simulink model "feeder_1_1_sm_feeder1"  (Simulink 9.2)
settings: Solver=ode4  StartTime=0.0  StopTime=inf  FixedStep=0.0001  RelTol=1e-3
PreLoadFcn:
  | Ts=100e-6;Core_Num = 0;
PostLoadFcn:
  | Ts=100e-6;Core_Num = 0;
InitFcn:
  | Ts=100e-6;Core_Num = 0;
undefined symbols (not defined in the file or in its folder): another_event_name, D11, Delta, my_event_name
libraries: powerlib x91, powerlib_meascontrol x28, simulink x9, opal_lib x3, artemis x2, rtio_generic_ethernet x1, rtio_opalrt_ml605ex1 x1, rtlab x1, rtio_spectracom x1
(part 1 of 2)
settings Model: ARTEMISmethode_block_infos=$$__separator__$$feeder_1_1_sm_feeder1/ARTEMIS Guide1$$__separator__$$  Creator=DETLDAQ  LastModifiedBy=DETLDAQ
settings OptimizationCC: BlockReduction=off  BooleanDataType=off  OptimizeBlockIOStorage=off  BufferReuse=off  GlobalBufferReuse=off  ExpressionFolding=off  LocalBlockOutputs=off  OptimizeDataStoreBuffers=off  BusAssignmentInplaceUpdate=off
settings DebuggingCC: SaveWithParameterizedLinksMsg=none  SignalResolutionControl=TryResolveAllWithWarning  MultiTaskDSMMsg=warning  MultiTaskCondExecSysMsg=none  FcnCallInpInsideContextMsg=error
settings HardwareCC: TargetUnknown=on
settings RTWCC: GenCodeOnly=on
settings GRTTargetCC: CombineOutputUpdateFcns=on  GRTInterface=off
settings SimscapeCC: SimscapeNormalizeSystem=off

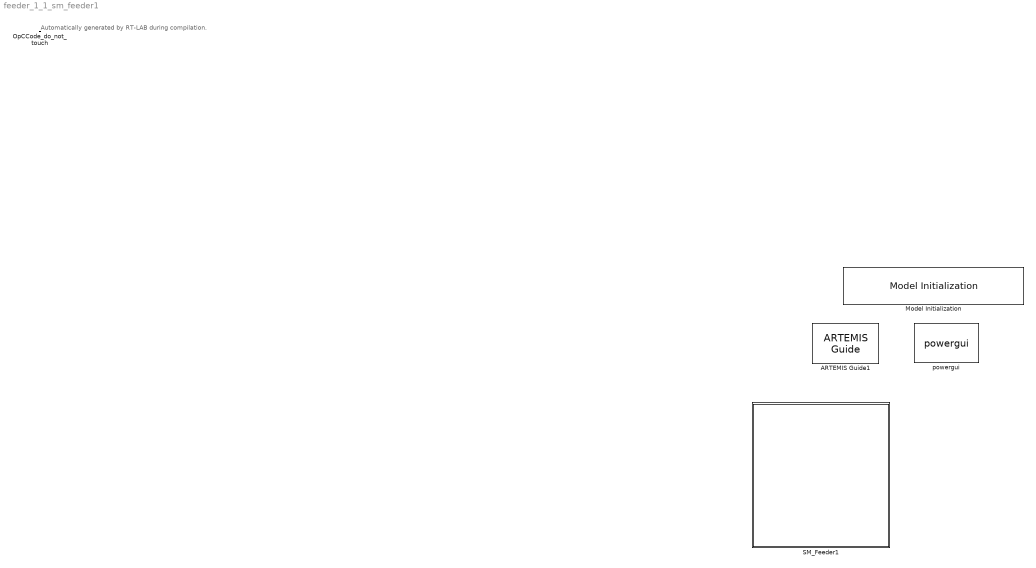
== system feeder_1_1_sm_feeder1 ==
  note: Automatically generated by RT-LAB during compilation.
  ARTEMIS Guide1 : artemis/ARTEMIS/ARTEMIS Guide  Tag=FTSSmethode_opal_4hx0r99  Description=5.0_z1  lock=on  Ts=Ts  opt=art5  dyna=off  nb_perm=4  RT_fullcomp=off  ssn=on  ssn_itvc=off  ssn_ivic=off  ssn_ext=off  ssn_solver=Backward Euler  ssn_impulse=off  ssn_quasimpulse=off  ssn_impulse_loop=5  paraExtinctionThy=off  Thy_Impulse=off  dtc=Off  dtc_opt=normal  ao=on  simtype=off  ct_mac=off  lin_mov=off  lsp=[0.001 2]  spike_skip=Disabled  dtc_extra=1  dtc_sws=normal  dtc_pied=0.5  SPSRulesBlock=SPSRules  tre=off  ctmm=off  LF=on  dpl_type=ARTEMiS DPL  rlc_type=off  custom_type=off  para=on  ssn_ImpulseLoopBlockedStateUpdate=5  ssn_mov_iter_number=5  ssn_switch_iter_number=5  ssn_nib_type_verify=on  ssn_use_lu=on  ssn_use_ldlt=off
  Model Initialization : artemis/Tools /Misc/Model Initialization  InitFcnX=Ts=100e-6;Core_Num = 0;  prel=on  posl=on  inif=on  strf=off
  OpCCode_do_not_touch : opal_lib/Communication/OpCCode  SystemSampleTime=-1
  SM_Feeder1 : Subsystem
  powergui : powerlib/powergui  SimulationMode=Discrete  SampleTime=0.0001  frequency=60  Iterations=50  frequencyindice=0  Pbase=100e6  ErrMax=0.0001  UnitsV=kV  UnitsW=MW  buscounter=0  FunctionMessages=off  echomessages=off  EnableUseOfTLC=off  CurrentSourceSwitches=off  DisableSnubberDevices=off  DisableRonSwitches=off  DisableVfSwitches=off  DisplayEquations=off  SolverType=Backward Euler  Interpol=off  ExternalGateDelay=off  methode=off  Ts=100  x0status=blocks  SPID=off  SwTol=0  HookPort=off  RestoreLinks=warning  ResistiveCurrentMeasurement=off  Frange=[0:2:500]  Ylog=off  Xlog=on  ShowGrid=off  save=off  variable=ZData  structure=0  ZoomFFT=off  StartTime=0.0  cycles=1  DisplayStyle=1  fundamental=60  FreqAxis=off  MaxFrequency=1000  frequencyindicesteady=1  RmsSteady=1  display=off

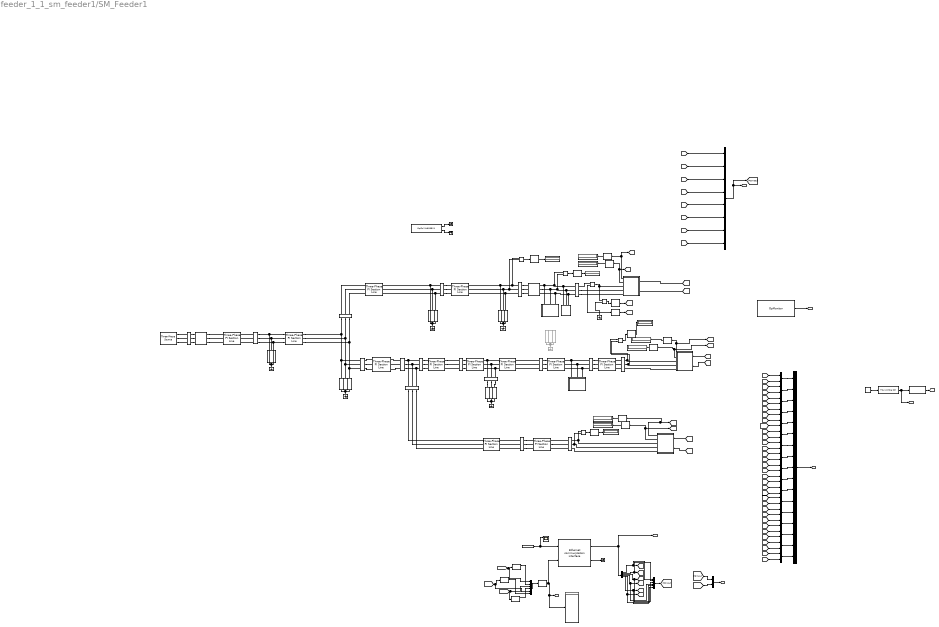
== system feeder_1_1_sm_feeder1/SM_Feeder1 ==
  note: included
  note: Included
  note: Included in SE
  note: Not include
  note: Not include in SE
  note: not include in SE
  Auxiliary Load : powerlib/Elements/Three-Phase Parallel RLC Load  LConnTagsString=A|B|C  Configuration=Y (grounded)  NominalVoltage=480  Vabc=[1e3 1e3 1e3]  Vabcp=[1e3 1e3 1e3]  NominalFrequency=60  UnbalancedPower=off  ActivePower=1  InductivePower=0  CapacitivePower=0  Pabc=[10e3 9e3 11e3]  QLabc=[100 90 110]  QCabc=[100 90 110]  Pabcp=[10e3 9e3 11e3]  QLabcp=[100 90 110]  QCabcp=[100 90 110]  Measurements=None  LoadType=constant Z
  Bus Creator : BusCreator  Inputs=17
  Constant8 : Constant
  Current Measurement : powerlib/Measurements/Current Measurement  PhasorSimulation=off  OutputType=Complex  PSBequivalent=0
  Demux1 : Demux  Outputs=6
  Display{,1,4..9,15..16} (10 alike) : Display
      Display15 settings: Format=bank
      Display4 settings: Format=bank
      Display5 settings: Format=bank
      Display7 settings: Format=bank
      Display8 settings: Format=bank
  Dynamic Load BCDC : Subsystem
  Dynamic Load Landfill : Subsystem
  Ethernet communication interface : rtio_generic_ethernet/Ethernet communication interface  ctrl_id=1  nbr_to_remote_endpoint=12  type_to_remote_endpoint=FLOAT  offset_to_remote_endpoint=0  swap_tx=on  nbr_from_remote_endpoint=6  type_from_remote_endpoint=FLOAT  offset_from_remote_endpoint=0  swap_rx=on  exe_name='AsyncEthernet'  nic_name='eth0'  protocol=TCP  tcp_mode=Client  port=6340  remote_ip='10.1.2.2'
  Ground{1..3,5,7..8} (6 alike) : powerlib/Elements/Ground  LConnTagsString=a
  Ground4 : powerlib/Elements/Ground  Commented=on  LConnTagsString=a
  IED1 : powerlib/Measurements/Three-Phase V-I Measurement  VoltageMeasurement=phase-to-ground  SetLabelV=on  LabelV=V_IED1  Vpu=off  VpuLL=off  CurrentMeasurement=yes  SetLabelI=on  LabelI=I_IED1  Ipu=off  Pbase=100e6  Vbase=500e3  OutputType=Complex  PhasorSimulation=off  PSBequivalent=0
  IED10 : powerlib/Measurements/Three-Phase V-I Measurement  VoltageMeasurement=phase-to-ground  SetLabelV=on  LabelV=V_IED10  Vpu=off  VpuLL=off  CurrentMeasurement=yes  SetLabelI=on  LabelI=I_IED10  Ipu=off  Pbase=100e6  Vbase=500e3  OutputType=Complex  PhasorSimulation=off  PSBequivalent=0
  IED11 : powerlib/Measurements/Three-Phase V-I Measurement  VoltageMeasurement=phase-to-ground  SetLabelV=on  LabelV=V_IED11  Vpu=off  VpuLL=off  CurrentMeasurement=yes  SetLabelI=on  LabelI=I_IED11  Ipu=off  Pbase=100e6  Vbase=500e3  OutputType=Complex  PhasorSimulation=off  PSBequivalent=0
  IED12 : powerlib/Measurements/Three-Phase V-I Measurement  VoltageMeasurement=phase-to-ground  SetLabelV=on  LabelV=V_IED12  Vpu=off  VpuLL=off  CurrentMeasurement=yes  SetLabelI=on  LabelI=I_IED12  Ipu=off  Pbase=100e6  Vbase=500e3  OutputType=Complex  PhasorSimulation=off  PSBequivalent=0
  IED13 : powerlib/Measurements/Three-Phase V-I Measurement  VoltageMeasurement=phase-to-ground  SetLabelV=on  LabelV=V_IED13  Vpu=off  VpuLL=off  CurrentMeasurement=yes  SetLabelI=on  LabelI=I_IED13  Ipu=off  Pbase=100e6  Vbase=500e3  OutputType=Complex  PhasorSimulation=off  PSBequivalent=0
  IED14 : powerlib/Measurements/Three-Phase V-I Measurement  VoltageMeasurement=phase-to-ground  SetLabelV=on  LabelV=V_IED14  Vpu=off  VpuLL=off  CurrentMeasurement=yes  SetLabelI=on  LabelI=I_IED14  Ipu=off  Pbase=100e6  Vbase=500e3  OutputType=Complex  PhasorSimulation=off  PSBequivalent=0
  IED15 : powerlib/Measurements/Three-Phase V-I Measurement  VoltageMeasurement=phase-to-ground  SetLabelV=on  LabelV=V_IED15  Vpu=off  VpuLL=off  CurrentMeasurement=yes  SetLabelI=on  LabelI=I_IED15  Ipu=off  Pbase=100e6  Vbase=500e3  OutputType=Complex  PhasorSimulation=off  PSBequivalent=0
  IED16 : powerlib/Measurements/Three-Phase V-I Measurement  VoltageMeasurement=phase-to-ground  SetLabelV=on  LabelV=V_IED16  Vpu=off  VpuLL=off  CurrentMeasurement=yes  SetLabelI=on  LabelI=I_IED16  Ipu=off  Pbase=100e6  Vbase=500e3  OutputType=Complex  PhasorSimulation=off  PSBequivalent=0
  IED17 : powerlib/Measurements/Three-Phase V-I Measurement  VoltageMeasurement=phase-to-ground  SetLabelV=on  LabelV=V_IED17  Vpu=off  VpuLL=off  CurrentMeasurement=yes  SetLabelI=on  LabelI=I_IED17  Ipu=off  Pbase=100e6  Vbase=500e3  OutputType=Complex  PhasorSimulation=off  PSBequivalent=0
  IED2 : powerlib/Measurements/Three-Phase V-I Measurement  VoltageMeasurement=phase-to-ground  SetLabelV=on  LabelV=V_IED2  Vpu=off  VpuLL=off  CurrentMeasurement=yes  SetLabelI=on  LabelI=I_IED2  Ipu=off  Pbase=100e6  Vbase=500e3  OutputType=Complex  PhasorSimulation=off  PSBequivalent=0
  IED3 : powerlib/Measurements/Three-Phase V-I Measurement  VoltageMeasurement=phase-to-ground  SetLabelV=on  LabelV=V_IED3  Vpu=off  VpuLL=off  CurrentMeasurement=yes  SetLabelI=on  LabelI=I_IED3  Ipu=off  Pbase=100e6  Vbase=500e3  OutputType=Complex  PhasorSimulation=off  PSBequivalent=0
  IED4 : powerlib/Measurements/Three-Phase V-I Measurement  VoltageMeasurement=phase-to-ground  SetLabelV=on  LabelV=V_IED4  Vpu=off  VpuLL=off  CurrentMeasurement=yes  SetLabelI=on  LabelI=I_IED4  Ipu=off  Pbase=100e6  Vbase=500e3  OutputType=Complex  PhasorSimulation=off  PSBequivalent=0
  IED5 : powerlib/Measurements/Three-Phase V-I Measurement  VoltageMeasurement=phase-to-ground  SetLabelV=on  LabelV=V_IED5  Vpu=off  VpuLL=off  CurrentMeasurement=yes  SetLabelI=on  LabelI=I_IED5  Ipu=off  Pbase=100e6  Vbase=500e3  OutputType=Complex  PhasorSimulation=off  PSBequivalent=0
  IED6 : powerlib/Measurements/Three-Phase V-I Measurement  VoltageMeasurement=phase-to-ground  SetLabelV=on  LabelV=V_IED6  Vpu=off  VpuLL=off  CurrentMeasurement=yes  SetLabelI=on  LabelI=I_IED6  Ipu=off  Pbase=100e6  Vbase=500e3  OutputType=Complex  PhasorSimulation=off  PSBequivalent=0
  IED7 : powerlib/Measurements/Three-Phase V-I Measurement  VoltageMeasurement=phase-to-ground  SetLabelV=on  LabelV=V_IED7  Vpu=off  VpuLL=off  CurrentMeasurement=yes  SetLabelI=on  LabelI=I_IED7  Ipu=off  Pbase=100e6  Vbase=500e3  OutputType=Complex  PhasorSimulation=off  PSBequivalent=0
  IED8 : powerlib/Measurements/Three-Phase V-I Measurement  VoltageMeasurement=phase-to-ground  SetLabelV=on  LabelV=V_IED8  Vpu=off  VpuLL=off  CurrentMeasurement=yes  SetLabelI=on  LabelI=I_IED8  Ipu=off  Pbase=100e6  Vbase=500e3  OutputType=Complex  PhasorSimulation=off  PSBequivalent=0
  IED9 : powerlib/Measurements/Three-Phase V-I Measurement  VoltageMeasurement=phase-to-ground  SetLabelV=on  LabelV=V_IED9  Vpu=off  VpuLL=off  CurrentMeasurement=yes  SetLabelI=on  LabelI=I_IED9  Ipu=off  Pbase=100e6  Vbase=500e3  OutputType=Complex  PhasorSimulation=off  PSBequivalent=0
  Line105 : powerlib/Elements/Three-Phase PI Section Line  LConnTagsString=a|b|c  RConnTagsString=A|B|C  Frequency=60  Resistances=[0.713799213 1.084564961]  Inductances=[0.001374518 0.004235717]  Capacitances=[1.12126E-07 1.12126E-07]  Length=3.436427976
      settings: SourceProductName=Simscape Power Systems
  Line135 : powerlib/Elements/Three-Phase PI Section Line  LConnTagsString=a|b|c  RConnTagsString=A|B|C  Frequency=60  Resistances=[0.437335958 0.80347769]  Inductances=[ 0.00135414 0.00422516]  Capacitances=[1.12126E-07 1.12126E-07]  Length=0.054899113
      settings: SourceProductName=Simscape Power Systems
  Line149 : powerlib/Elements/Three-Phase PI Section Line  LConnTagsString=a|b|c  RConnTagsString=A|B|C  Frequency=60  Resistances=[0.080380577 0.200459318]  Inductances=[0.000297632 0.000175795]  Capacitances=[1.12126E-07 1.12126E-07]  Length=0.001045348
      settings: SourceProductName=Simscape Power Systems
  Line150 : powerlib/Elements/Three-Phase PI Section Line  LConnTagsString=a|b|c  RConnTagsString=A|B|C  Frequency=60  Resistances=[0.076844259 0.363286089]  Inductances=[0.000938984 0.003273312]  Capacitances=[1.12126E-07 1.12126E-07]  Length=3.569857224
      settings: SourceProductName=Simscape Power Systems
  Line164 : powerlib/Elements/Three-Phase PI Section Line  LConnTagsString=a|b|c  RConnTagsString=A|B|C  Frequency=60  Resistances=[0.104986877 0.326771654]  Inductances=[0.000315038 0.000223659]  Capacitances=[1.12126E-07 1.12126E-07]  Length=0.024037250
      settings: SourceProductName=Simscape Power Systems
  Line167 : powerlib/Elements/Three-Phase PI Section Line  LConnTagsString=a|b|c  RConnTagsString=A|B|C  Frequency=60  Resistances=[0.146325459 0.420275591]  Inductances=[0.001054767 0.003564625]  Capacitances=[1.12126E-07 1.12126E-07]  Length=0.039662466
      settings: SourceProductName=Simscape Power Systems
  Line188 : powerlib/Elements/Three-Phase PI Section Line  LConnTagsString=a|b|c  RConnTagsString=A|B|C  Frequency=60  Resistances=[0.074475066 0.348425197]  Inductances=[0.000982535 0.003492392]  Capacitances=[1.12126E-07 1.12126E-07]  Length=0.354198631
      settings: SourceProductName=Simscape Power Systems
  Line196 : powerlib/Elements/Three-Phase PI Section Line  LConnTagsString=a|b|c  RConnTagsString=A|B|C  Frequency=60  Resistances=[0.1820739 0.3053387]  Inductances=[0.000581495 0.000514283]  Capacitances=[3.41761e-8 3.4176e-8]  Length=0.029452870
      settings: SourceProductName=Simscape Power Systems
  Line4 : powerlib/Elements/Three-Phase PI Section Line  LConnTagsString=a|b|c  RConnTagsString=A|B|C  Frequency=60  Resistances=[8.150387E-02 0.348876969]  Inductances=[0.000906839 0.003088814]  Capacitances=[1.12126E-07 1.12126E-07]  Length=0.314096400
      settings: SourceProductName=Simscape Power Systems
  Line59 : powerlib/Elements/Three-Phase PI Section Line  LConnTagsString=a|b|c  RConnTagsString=A|B|C  Frequency=60  Resistances=[0.074475066 0.348425197]  Inductances=[0.000982535 0.003492393]  Capacitances=[1.12126E-07 1.12126E-07]  Length=1.094945842
      settings: SourceProductName=Simscape Power Systems
  Line88 : powerlib/Elements/Three-Phase PI Section Line  LConnTagsString=a|b|c  RConnTagsString=A|B|C  Frequency=60  Resistances=[7.447507E-02 0.348425197]  Inductances=[0.000982535 0.003492393]  Capacitances=[1.12126E-07 1.12126E-07]  Length=0.079929441
      settings: SourceProductName=Simscape Power Systems
  Line97 : powerlib/Elements/Three-Phase PI Section Line  LConnTagsString=a|b|c  RConnTagsString=A|B|C  Frequency=60  Resistances=[7.447507E-02 0.348425197]  Inductances=[0.000982535 0.003492393]  Capacitances=[1.12126E-07 1.12126E-07]  Length=0.080325681
      settings: SourceProductName=Simscape Power Systems
  Mux{1,3..4,6..19,34} (18 alike) : Mux  Inputs=2
  Mux2 : Mux  Inputs=8
  Mux20 : Mux  Inputs=6
  Mux5 : Mux  Inputs=6
  OpCtrl ML605EX1 : rtio_opalrt_ml605ex1/OpCtrl ML605EX1  CtrlName='ML605EX1 Ctrl'  boardid=0  BitstreamFilename=ML605_2-EX-0029-2_2_6_61-32Aio_32DioSelectable-01-01.bin  numconfig=-1  mode=Master  externalClock=off  decimRtsi=0  calibIO=off  SampleTime=0  loadinport=-1
  OpMonitor : rtlab/Monitoring/OpMonitor  compute_time=off  real_step=off  idle_time=off  nb_overruns=on  user_time=off  user_name=my_event_name,another_event_name
  PLL (3ph) : powerlib_meascontrol/PLL/PLL (3ph)  Fmin=45  Par_Init=[0, 60]  ParK=[180, 3200, 1]  TcD=1e-4  MaxRateChangeFreq=12  FilterCutOffFreq=25  Ts=0  AGC=on
  PLL (3ph)1 : powerlib_meascontrol/PLL/PLL (3ph)  Fmin=45  Par_Init=[0, 60]  ParK=[180, 3200, 1]  TcD=1e-4  MaxRateChangeFreq=12  FilterCutOffFreq=25  Ts=0  AGC=on
  PLL (3ph)2 : powerlib_meascontrol/PLL/PLL (3ph)  Fmin=45  Par_Init=[0, 60]  ParK=[180, 3200, 1]  TcD=1e-4  MaxRateChangeFreq=12  FilterCutOffFreq=25  Ts=0  AGC=on
  PLL power injector : Subsystem  mask{ratedP=258*1000, ratedV=480, KP_I=2, KI_I=20, Res=0.00893, Ind=1.895e-3}
      mask prompts: ratedP "Rated Power (VA)"; ratedV "Rated Voltage (Vrms)"; KP_I "KP of Current Regulator"; KI_I "KI of current regulator"; Res "Ri (ohms)"; Ind "Li (Henrys)"
      mask init:
      | Sb = ratedP;
      | Vb = ratedV*sqrt(2)/sqrt(3);
      | Wb = 2*pi*60;
      | Ib = Sb*sqrt(2)/ratedV/sqrt(3);
      | Zb = Vb/Ib;
      | Lb = Zb/Wb;
      | 
      | Ri = Res;
      | Li = Ind;
      | Ri_pu = Ri/Zb;
      | Li_pu = Li/Lb;
      | 
      | KP = KP_I;
      | KI = KI_I;
  PLL power injector1 : Subsystem  mask{ratedP=10000000, ratedV=12470, KP_I=2, KI_I=20, Res=0.01555, Ind=3.3e-3}
      mask prompts: ratedP "Rated Power (VA)"; ratedV "Rated Voltage (Vrms)"; KP_I "KP of Current Regulator"; KI_I "KI of current regulator"; Res "Ri (ohms)"; Ind "Li (Henrys)"
      mask init:
      | Sb = ratedP;
      | Vb = ratedV*sqrt(2)/sqrt(3);
      | Wb = 2*pi*60;
      | Ib = Sb*sqrt(2)/ratedV/sqrt(3);
      | Zb = Vb/Ib;
      | Lb = Zb/Wb;
      | 
      | Ri = Res;
      | Li = Ind;
      | Ri_pu = Ri/Zb;
      | Li_pu = Li/Lb;
      | 
      | KP = KP_I;
      | KI = KI_I;
  PLL power injector2 : Subsystem  mask{ratedP=10000000, ratedV=12470, KP_I=2, KI_I=20, Res=0.1555, Ind=0.033}
      mask prompts: ratedP "Rated Power (VA)"; ratedV "Rated Voltage (Vrms)"; KP_I "KP of Current Regulator"; KI_I "KI of current regulator"; Res "Ri (ohms)"; Ind "Li (Henrys)"
      mask init:
      | Sb = ratedP;
      | Vb = ratedV*sqrt(2)/sqrt(3);
      | Wb = 2*pi*60;
      | Ib = Sb*sqrt(2)/ratedV/sqrt(3);
      | Zb = Vb/Ib;
      | Lb = Zb/Wb;
      | 
      | Ri = Res;
      | Li = Ind;
      | Ri_pu = Ri/Zb;
      | Li_pu = Li/Lb;
      | 
      | KP = KP_I;
      | KI = KI_I;
  Pulse input : DiscretePulseGenerator  Period=round(1/Ts)  SampleTime=Ts
  RMS{,1..6,11..15} (12 alike) : powerlib_meascontrol/Measurements/RMS  TrueRMS=on  Freq=60  RMSInit=120  Ts=Ts
  RMS28 : powerlib_meascontrol/Measurements/RMS  TrueRMS=on  Freq=60  RMSInit=480  Ts=Ts
  Scope : Scope  NumInputPorts=2
  Series  Load1 : powerlib/Elements/Series RLC Load  LConnTagsString=a  RConnTagsString=__new0  NominalVoltage=7199.557857  NominalFrequency=60  ActivePower=2670.415479  InductivePower=302.451287  CapacitivePower=0  Setx0=off  InitialVoltage=0  SetiL0=off  InitialCurrent=0  Measurements=None  LoadType=constant PQ
  Series  Load10 : powerlib/Elements/Series RLC Load  Commented=on  LConnTagsString=a  RConnTagsString=__new0  NominalVoltage=480  NominalFrequency=60  ActivePower=25500  InductivePower=19200  CapacitivePower=0  Setx0=off  InitialVoltage=0  SetiL0=off  InitialCurrent=0  Measurements=None  LoadType=constant PQ
  Series  Load11 : powerlib/Elements/Series RLC Load  Commented=on  LConnTagsString=a  RConnTagsString=__new0  NominalVoltage=480  NominalFrequency=60  ActivePower=25500  InductivePower=19200  CapacitivePower=0  Setx0=off  InitialVoltage=0  SetiL0=off  InitialCurrent=0  Measurements=None  LoadType=constant PQ
  Series  Load12 : powerlib/Elements/Series RLC Load  Commented=on  LConnTagsString=a  RConnTagsString=__new0  NominalVoltage=480  NominalFrequency=60  ActivePower=25500  InductivePower=19200  CapacitivePower=0  Setx0=off  InitialVoltage=0  SetiL0=off  InitialCurrent=0  Measurements=None  LoadType=constant PQ
  Series  Load13 : powerlib/Elements/Series RLC Load  LConnTagsString=a  RConnTagsString=__new0  NominalVoltage=7199.557857  NominalFrequency=60  ActivePower=118930.1571  InductivePower=12605.38342  CapacitivePower=0  Setx0=off  InitialVoltage=0  SetiL0=off  InitialCurrent=0  Measurements=None  LoadType=constant PQ
  Series  Load14 : powerlib/Elements/Series RLC Load  LConnTagsString=a  RConnTagsString=__new0  NominalVoltage=7199.557857  NominalFrequency=60  ActivePower=107384.1981  InductivePower=11558.83111  CapacitivePower=0  Setx0=off  InitialVoltage=0  SetiL0=off  InitialCurrent=0  Measurements=None  LoadType=constant PQ
  Series  Load15 : powerlib/Elements/Series RLC Load  LConnTagsString=a  RConnTagsString=__new0  NominalVoltage=7199.557857  NominalFrequency=60  ActivePower=108561.8938  InductivePower=11911.28039  CapacitivePower=0  Setx0=off  InitialVoltage=0  SetiL0=off  InitialCurrent=0  Measurements=None  LoadType=constant PQ
  Series  Load16 : powerlib/Elements/Series RLC Load  LConnTagsString=a  RConnTagsString=__new0  NominalVoltage=7199.557857  NominalFrequency=60  ActivePower=116317.6881  InductivePower=25615.54001  CapacitivePower=0  Setx0=off  InitialVoltage=0  SetiL0=off  InitialCurrent=0  Measurements=None  LoadType=constant PQ
  Series  Load17 : powerlib/Elements/Series RLC Load  LConnTagsString=a  RConnTagsString=__new0  NominalVoltage=7199.557857  NominalFrequency=60  ActivePower=97118.47107  InductivePower=22060.3874  CapacitivePower=0  Setx0=off  InitialVoltage=0  SetiL0=off  InitialCurrent=0  Measurements=None  LoadType=constant PQ
  Series  Load18 : powerlib/Elements/Series RLC Load  LConnTagsString=a  RConnTagsString=__new0  NominalVoltage=7199.557857  NominalFrequency=60  ActivePower=100579.6302  InductivePower=22407.05615  CapacitivePower=0  Setx0=off  InitialVoltage=0  SetiL0=off  InitialCurrent=0  Measurements=None  LoadType=constant PQ
  Series  Load19 : powerlib/Elements/Series RLC Load  LConnTagsString=a  RConnTagsString=__new0  NominalVoltage=12470  NominalFrequency=60  ActivePower=0  InductivePower=0  CapacitivePower=1800000  Setx0=off  InitialVoltage=0  SetiL0=off  InitialCurrent=0  Measurements=None  LoadType=constant Z
  Series  Load2 : powerlib/Elements/Series RLC Load  LConnTagsString=a  RConnTagsString=__new0  NominalVoltage=7199.557857  NominalFrequency=60  ActivePower=0  InductivePower=3.438665  CapacitivePower=0  Setx0=off  InitialVoltage=0  SetiL0=off  InitialCurrent=0  Measurements=None  LoadType=constant PQ
  Series  Load20 : powerlib/Elements/Series RLC Load  LConnTagsString=a  RConnTagsString=__new0  NominalVoltage=12470  NominalFrequency=60  ActivePower=0  InductivePower=0  CapacitivePower=1800000  Setx0=off  InitialVoltage=0  SetiL0=off  InitialCurrent=0  Measurements=None  LoadType=constant Z
  Series  Load21 : powerlib/Elements/Series RLC Load  LConnTagsString=a  RConnTagsString=__new0  NominalVoltage=12470  NominalFrequency=60  ActivePower=0  InductivePower=0  CapacitivePower=1800000  Setx0=off  InitialVoltage=0  SetiL0=off  InitialCurrent=0  Measurements=None  LoadType=constant Z
  Series  Load3 : powerlib/Elements/Series RLC Load  LConnTagsString=a  RConnTagsString=__new0  NominalVoltage=7199.557857  NominalFrequency=60  ActivePower=3860.344758  InductivePower=489.471522  CapacitivePower=0  Setx0=off  InitialVoltage=0  SetiL0=off  InitialCurrent=0  Measurements=None  LoadType=constant PQ
  Series  Load4 : powerlib/Elements/Series RLC Load  LConnTagsString=a  RConnTagsString=__new0  NominalVoltage=7199.557857  NominalFrequency=60  ActivePower=393.998726  InductivePower=154.409997  CapacitivePower=0  Setx0=off  InitialVoltage=0  SetiL0=off  InitialCurrent=0  Measurements=None  LoadType=constant PQ
  Series  Load5 : powerlib/Elements/Series RLC Load  LConnTagsString=a  RConnTagsString=__new0  NominalVoltage=7199.557857  NominalFrequency=60  ActivePower=28.182185  InductivePower=0  CapacitivePower=8.948845  Setx0=off  InitialVoltage=0  SetiL0=off  InitialCurrent=0  Measurements=None  LoadType=constant PQ
  Series  Load6 : powerlib/Elements/Series RLC Load  LConnTagsString=a  RConnTagsString=__new0  NominalVoltage=7199.557857  NominalFrequency=60  ActivePower=2288.289329  InductivePower=413.71859  CapacitivePower=0  Setx0=off  InitialVoltage=0  SetiL0=off  InitialCurrent=0  Measurements=None  LoadType=constant PQ
  TSync PCIe Ctrl1 : rtio_spectracom/TSync PCIe Ctrl  devIx=0  holdover_timeout=5  timestamp_en=on  set_time_en=off  ts_wo_sync_opt=Simulation time
  Terminator1 : Terminator
  Terminator2 : Terminator
  Terminator3 : Terminator
  Three-Phase Transformer (Two Windings) : powerlib/Elements/Three-Phase Transformer (Two Windings)  Winding1Connection=Delta (D11)  Winding2Connection=Yg  CoreType=Three single-phase transformers  SetSaturation=off  Hysteresis=off  DataFile='hysteresis'  SetInitialFlux=off  Measurements=None  UNITS=pu  NominalPower=[30000e3 , 60 ]  Winding1=[ 115e3 , 0.0005 , 0.07755]  Winding2=[ 12.47e3, 0.0005 ,0.07755 ]  Rm=200  Lm=200  L0=0.5  Saturation=[ 0,0 ; 0.0024,1.2 ; 1.0,1.52 ]  InitialFluxes=[ 0.8 , -0.8 , 0.7 ]  MoreParameters=off  BreakLoop=off  DataType=off  TransfoNumber=1
  Three-Phase Transformer (Two Windings)5 : powerlib/Elements/Three-Phase Transformer (Two Windings)  Winding1Connection=Yg  Winding2Connection=Yg  CoreType=Three single-phase transformers  SetSaturation=off  Hysteresis=off  DataFile='hysteresis'  SetInitialFlux=off  Measurements=Winding voltages  UNITS=pu  NominalPower=[500e3 , 60 ]  Winding1=[ 12.47e3 , 0.002 , 0.035 ]  Winding2=[ 480 , 0.002 ,0.035 ]  Rm=500  Lm=500  L0=0.5  Saturation=[ 0,0 ; 0.0024,1.2 ; 1.0,1.52 ]  InitialFluxes=[ 0.8 , -0.8 , 0.7 ]  MoreParameters=off  BreakLoop=off  DataType=off  TransfoNumber=1
  Three-Phase Source : powerlib/Electrical Sources/Three-Phase Source  InternalConnection=Yg  VoltagePhases=off  Voltage=(115000)*1.0001  PhaseAngle=0  Voltage_phases=[25e3 25e3 25e3]/sqrt(3)  PhaseAngles_phases=[0 -120 +120]  Frequency=60  NonIdealSource=on  SpecifyImpedance=off  Resistance=1.5  Inductance=0.02122065907  ShortCircuitLevel=1624.8e6  BaseVoltage=115e3  XRratio=5  BusType=swing  Pref=0  Qref=0  Prefabc=[10e3, 10e3, 10e3]  Qrefabc=[0, 0, 0]  Qmin=-inf  Qmax=inf
  Timestamp selector : Subsystem
  V : Display
  Voltage Measurement{,1..4} (5 alike) : powerlib/Measurements/Voltage Measurement  PhasorSimulation=off  OutputType=Complex  PSBequivalent=0
  rtlab_send_subsystem : Subsystem  Priority=-100
      mask Display: text(0,0,'');
  tag scope: PQinput=global, rtlab_send_1=global, rtlab_send_2=global, rtlab_send_3=global, rtlab_send_4=global, rtlab_send_5=global, rtlab_send_6=global, rtlab_send_7=global, rtlab_send_8=global
  wires:
  OpCtrl ML605EX1/1 -> Terminator1/1
  OpCtrl ML605EX1/2 -> Terminator3/1
  [P1] -> Mux2/1
  [Q1] -> Mux2/2
  [P2] -> Mux2/3
  [Q2] -> Mux2/4
  [P3] -> Mux2/5
  [Q3] -> Mux2/6
  [V_IED1] -> Mux4/1
  [I_IED1] -> Mux4/2
  [V_IED2] -> Mux6/1
  [I_IED2] -> Mux6/2
  [V_IED3] -> Mux7/1
  [I_IED3] -> Mux7/2
  [V_IED5] -> Mux9/1
  [I_IED5] -> Mux9/2
  [V_IED6] -> Mux10/1
  [I_IED6] -> Mux10/2
  [V_IED7] -> Mux11/1
  [I_IED7] -> Mux11/2
  [V_IED8] -> Mux12/1
  [I_IED8] -> Mux12/2
  [V_IED10] -> Mux13/1
  [I_IED10] -> Mux13/2
  [V_IED11] -> Mux14/1
  [I_IED11] -> Mux14/2
  [V_IED12] -> Mux15/1
  [I_IED12] -> Mux15/2
  [V_IED13] -> Mux16/1
  [I_IED13] -> Mux16/2
  [V_IED14] -> Mux17/1
  [I_IED14] -> Mux17/2
  [V_IED15] -> Mux18/1
  [I_IED15] -> Mux18/2
  [V_IED9] -> Mux19/1
  [I_IED9] -> Mux19/2
  OpMonitor/1 -> [rtlab_send_2]
  Mux4/1 -> Bus Creator/1
  Mux6/1 -> Bus Creator/2
  Mux7/1 -> Bus Creator/3
  Mux8/1 -> Bus Creator/4
  Mux9/1 -> Bus Creator/5
  Mux10/1 -> Bus Creator/6
  Mux11/1 -> Bus Creator/7
  Mux12/1 -> Bus Creator/8
  Mux19/1 -> Bus Creator/9
  Mux13/1 -> Bus Creator/10
  Mux14/1 -> Bus Creator/11
  Mux15/1 -> Bus Creator/12
  Mux16/1 -> Bus Creator/13
  Mux17/1 -> Bus Creator/14
  Mux18/1 -> Bus Creator/15
  Constant8/1 -> TSync PCIe Ctrl1/1
  Timestamp selector/1(ts_out) -> [rtlab_send_4]
  TSync PCIe Ctrl1/1 -> [rtlab_send_5], Timestamp selector/1(ts_in)
  [V_IED16] -> Mux3/1
  [I_IED16] -> Mux3/2
  [V_IED17] -> Mux34/1
  [I_IED17] -> Mux34/2
  Mux3/1 -> Bus Creator/16
  Mux34/1 -> Bus Creator/17
  Bus Creator/1 -> [rtlab_send_3]
  [V_IED4] -> Mux8/1
  [I_IED4] -> Mux8/2
  RMS/1 -> Display/1
  Voltage Measurement/1 -> RMS/1
  RMS1/1 -> Display1/1
  Voltage Measurement1/1 -> RMS1/1
  RMS2/1 -> Display4/1
  Voltage Measurement2/1 -> RMS2/1
  RMS3/1 -> Display7/1
  Voltage Measurement3/1 -> RMS3/1
  PLL power injector/2(Q_OUT) -> [Q1], RMS15/1
  PLL power injector1/2(Q_OUT) -> [Q3], RMS12/1
  PLL power injector/1(P_OUT) -> [P1], RMS14/1
  PLL power injector1/1(P_OUT) -> [P3], RMS13/1
  PLL power injector2/2(Q_OUT) -> [Q2], RMS11/1
  PLL power injector2/1(P_OUT) -> [P2], RMS4/1
  RMS4/1 -> Display8/1
  RMS11/1 -> Display9/1
  RMS12/1 -> Display6/1
  RMS13/1 -> Display5/1
  RMS14/1 -> Display15/1
  RMS15/1 -> Display16/1
  Demux1/1 -> Mux20/1, [P1in]
  Demux1/2 -> Mux20/2, [Q1in]
  Demux1/3 -> Mux20/3, [P2in]
  Demux1/4 -> Mux20/4, [Q2in]
  Demux1/5 -> Mux20/5, [P3in]
  Demux1/6 -> Mux20/6, [Q3in]
  [V_IED6] -> PLL (3ph)/1, Mux5/1
  Mux5/1 -> RMS28/1
  [P1in] -> PLL power injector/1(P_ref)
  [Q1in] -> PLL power injector/2("Q_ref ")
  [V_IED9] -> Mux5/3, PLL (3ph)2/1
  [V_IED14] -> Mux5/5, PLL (3ph)1/1
  PLL (3ph)/1 -> Mux5/2
  Ethernet communication interface/1 -> Demux1/1, [rtlab_send_6]
  Pulse input/1 -> Scope/1, Ethernet communication interface/1
  Ethernet communication interface/2 -> Terminator2/1
  RMS28/1 -> Ethernet communication interface/2, V/1, [rtlab_send_7]
  [PQinput] -> Mux1/1
  Mux2/1 -> [PQmeas], [rtlab_send_1]
  [PQmeas] -> Mux1/2
  Mux1/1 -> [rtlab_send_8]
  Mux20/1 -> [PQinput]
  Voltage Measurement4/1 -> RMS5/1
  Current Measurement/1 -> RMS6/1
  [RMSV] -> Mux2/7
  [RMSI] -> Mux2/8
  RMS5/1 -> [RMSV]
  RMS6/1 -> [RMSI]
  [P2in] -> PLL power injector2/1(P_ref)
  [Q2in] -> PLL power injector2/2("Q_ref ")
  [P3in] -> PLL power injector1/1(P_ref)
  [Q3in] -> PLL power injector1/2("Q_ref ")
  PLL (3ph)2/1 -> Mux5/4
  PLL (3ph)1/1 -> Mux5/6
  connections:
  Line135/RConn1 -- Series  Load17/LConn1 -- IED4/LConn1
  Line135/RConn2 -- Series  Load18/LConn1 -- IED4/LConn2
  Line135/RConn3 -- Series  Load16/LConn1 -- IED4/LConn3
  IED17/LConn1 -- IED7/LConn1 -- IED16/LConn1
  IED16/LConn2 -- IED7/LConn2 -- IED17/LConn2
  IED16/LConn3 -- IED7/LConn3 -- IED17/LConn3
  IED13/LConn3 -- Dynamic Load BCDC/LConn3 -- Line4/RConn3
  Line97/RConn2 -- Line88/LConn2 -- IED11/LConn2
  Line97/RConn1 -- Line88/LConn1 -- IED11/LConn1
  IED11/LConn3 -- Line97/RConn3 -- Line88/LConn3
  IED13/LConn1 -- Dynamic Load BCDC/LConn1 -- Line4/RConn1
  IED13/LConn2 -- Dynamic Load BCDC/LConn2 -- Line4/RConn2
  Line105/RConn1 -- Series  Load14/LConn1 -- IED5/LConn1 -- Voltage Measurement1/LConn1
  Line105/RConn2 -- Series  Load15/LConn1 -- IED5/LConn2 -- Voltage Measurement1/LConn2
  Line105/RConn3 -- Series  Load13/LConn1 -- IED5/LConn3
  Voltage Measurement/LConn2 -- Auxiliary Load/LConn2 -- IED6/LConn2 -- Dynamic Load Landfill/LConn2 -- Three-Phase Transformer (Two Windings)5/RConn2
  IED6/LConn3 -- Auxiliary Load/LConn3 -- Dynamic Load Landfill/LConn3 -- Three-Phase Transformer (Two Windings)5/RConn3
  Auxiliary Load/LConn1 -- IED6/LConn1 -- Voltage Measurement/LConn1 -- Dynamic Load Landfill/LConn1 -- Three-Phase Transformer (Two Windings)5/RConn1
  Series  Load1/RConn1 -- Series  Load2/RConn1 -- Series  Load3/RConn1 -- Ground1/LConn1
  Series  Load6/RConn1 -- Series  Load5/RConn1 -- Ground2/LConn1 -- Series  Load4/RConn1
  Series  Load12/RConn1 -- Ground4/LConn1 -- Series  Load10/RConn1 -- Series  Load11/RConn1
  Series  Load15/RConn1 -- Series  Load14/RConn1 -- Series  Load13/RConn1 -- Ground5/LConn1
  Series  Load18/RConn1 -- Series  Load17/RConn1 -- Ground7/LConn1 -- Series  Load16/RConn1
  Series  Load21/RConn1 -- Series  Load19/RConn1 -- Series  Load20/RConn1 -- Ground8/LConn1
  Voltage Measurement2/LConn2 -- IED14/RConn2 -- PLL power injector1/RConn2
  Voltage Measurement2/LConn1 -- IED14/RConn1 -- PLL power injector1/RConn1
  Voltage Measurement3/LConn1 -- IED9/RConn1 -- PLL power injector2/RConn1
  Voltage Measurement3/LConn2 -- IED9/RConn2 -- PLL power injector2/RConn2
  Series  Load5/LConn1 -- IED3/LConn1 -- Line150/RConn1 -- IED15/LConn1
  Series  Load6/LConn1 -- IED3/LConn2 -- Line150/RConn2 -- IED15/LConn2
  Series  Load4/LConn1 -- IED3/LConn3 -- Line150/RConn3 -- IED15/LConn3
  Line150/LConn1 -- IED2/LConn1 -- Series  Load2/LConn1
  Line150/LConn2 -- IED2/LConn2 -- Series  Load3/LConn1
  Line150/LConn3 -- IED2/LConn3 -- Series  Load1/LConn1
  IED1/RConn3 -- Three-Phase Transformer (Two Windings)/LConn3
  IED2/RConn3 -- Line149/RConn3
  IED1/RConn2 -- Three-Phase Transformer (Two Windings)/LConn2
  IED11/RConn2 -- Series  Load21/LConn1
  IED15/RConn2 -- Line135/LConn2
  Three-Phase Transformer (Two Windings)/RConn1 -- Line149/LConn1
  PLL power injector1/RConn3 -- IED14/RConn3
  IED3/RConn1 -- Line59/LConn1
  IED3/RConn3 -- Line59/LConn3
  IED6/RConn3 -- PLL power injector/RConn3
  PLL power injector2/RConn3 -- IED9/RConn3
  Three-Phase Transformer (Two Windings)/RConn3 -- Line149/LConn3
  IED15/RConn1 -- Line135/LConn1
  IED3/RConn2 -- Line59/LConn2
  IED6/RConn2 -- PLL power injector/RConn2
  IED2/RConn1 -- Line149/RConn1
  IED15/RConn3 -- Line135/LConn3
  Three-Phase Transformer (Two Windings)/RConn2 -- Line149/LConn2
  IED2/RConn2 -- Line149/RConn2
  IED11/RConn3 -- Series  Load19/LConn1
  IED13/RConn1 -- Line164/LConn1
  IED12/RConn2 -- Line4/LConn2
  IED11/RConn1 -- Series  Load20/LConn1
  IED14/LConn3 -- Line164/RConn3
  IED12/LConn1 -- Line88/RConn1
  IED12/RConn3 -- Line4/LConn3
  IED14/LConn2 -- Line164/RConn2
  IED7/RConn2 -- Line59/RConn2
  IED9/LConn1 -- Line196/RConn1
  IED7/RConn3 -- Line59/RConn3
  IED17/RConn1 -- Line188/LConn1
  IED17/RConn2 -- Line188/LConn2
  IED5/RConn1 -- Three-Phase Transformer (Two Windings)5/LConn1
  IED9/LConn3 -- Line196/RConn3
  Line188/RConn2 -- IED10/LConn2
  IED7/RConn1 -- Line59/RConn1
  IED13/RConn3 -- Line164/LConn3
  IED4/RConn3 -- Line105/LConn3
  IED16/RConn1 -- Line167/LConn1
  IED8/LConn3 -- Line167/RConn3
  IED10/RConn3 -- Line97/LConn3
  Line196/RConn2 -- IED9/LConn2
  IED17/RConn3 -- Line188/LConn3
  IED1/RConn1 -- Three-Phase Transformer (Two Windings)/LConn1
  IED10/RConn2 -- Line97/LConn2
  IED12/RConn1 -- Line4/LConn1
  IED5/RConn2 -- Three-Phase Transformer (Two Windings)5/LConn2
  IED16/RConn3 -- Line167/LConn3
  IED8/RConn2 -- Line196/LConn2
  IED5/RConn3 -- Three-Phase Transformer (Two Windings)5/LConn3
  IED10/LConn3 -- Line188/RConn3
  IED4/RConn1 -- Line105/LConn1
  IED8/RConn1 -- Line196/LConn1
  IED8/LConn1 -- Line167/RConn1
  IED12/LConn2 -- Line88/RConn2
  IED12/LConn3 -- Line88/RConn3
  IED10/RConn1 -- Line97/LConn1
  IED14/LConn1 -- Line164/RConn1
  IED8/RConn3 -- Line196/LConn3
  IED13/RConn2 -- Line164/LConn2
  IED4/RConn2 -- Line105/LConn2
  IED8/LConn2 -- Line167/RConn2
  Line188/RConn1 -- IED10/LConn1
  IED16/RConn2 -- Line167/LConn2
  Voltage Measurement4/LConn1 -- Current Measurement/LConn1 -- PLL power injector/RConn1
  Three-Phase Source/RConn1 -- IED1/LConn1
  Three-Phase Source/RConn2 -- IED1/LConn2
  Three-Phase Source/RConn3 -- IED1/LConn3
  Ground3/LConn1 -- Voltage Measurement4/LConn2
  Current Measurement/RConn1 -- IED6/RConn1

== system feeder_1_1_sm_feeder1/SM_Feeder1/Dynamic Load BCDC ==
  Clock1 : Clock
  Reactive Power : Lookup_n-D  NumberOfTableDimensions=1  BreakpointsForDimension1=|  Table=|  ExtrapMethod=Clip  InternalRulePriority=Speed  RndMeth=Simplest  InputSameDT=on
      BreakpointsForDimension1=|
      | [0
      | 900
      | 1800
      | 2700
      | 3600
      | 4500
      | 5400
      | 6300
      | 7200
      | 8100
      | 9000
      | 9900
      | 10800
      | 11700
      | 12600
      | 13500
      | 14400
      | 15300
      | 16200
      | 17100
      | 18000
      | 18900
      | 19800
      | 20700
      | 21600
      | ]
      Table=|
      | [1227960
      | 1219320
      | 1242540
      | 1298700
      | 1272240
      | 1207980
      | 1340280
      | 1339200
      | 1373220
      | 1369440
      | 1350540
      | 1378620
      | 1290600
      | 1243620
      | 1319760
      | 1482300
      | 1488780
      | 1369440
      | 1368360
      | 1327320
      | 1350000
      | 1373760
      | 1414800
      | 1366200
      | 1454220
      | ]
  Real Power : Lookup_n-D  NumberOfTableDimensions=1  BreakpointsForDimension1=|  Table=|  ExtrapMethod=Clip  InternalRulePriority=Speed  RndMeth=Simplest  InputSameDT=on
      BreakpointsForDimension1=|
      | [0
      | 900
      | 1800
      | 2700
      | 3600
      | 4500
      | 5400
      | 6300
      | 7200
      | 8100
      | 9000
      | 9900
      | 10800
      | 11700
      | 12600
      | 13500
      | 14400
      | 15300
      | 16200
      | 17100
      | 18000
      | 18900
      | 19800
      | 20700
      | 21600
      | ]
      Table=|
      | [1087020
      | 1058940
      | 916380
      | 919620
      | 986580
      | 981720
      | 882360
      | 884520
      | 921240
      | 957420
      | 1030320
      | 865620
      | 1218780
      | 1271700
      | 1136700
      | 1005480
      | 1060560
      | 1320300
      | 1183140
      | 1209600
      | 1216620
      | 1095120
      | 1131300
      | 1144260
      | 983880
      | ]
  Three-Phase Dynamic Load : powerlib/Elements/Three-Phase Dynamic Load  NominalVoltage=[ 480e3 60 ]  ActiveReactivePowers=[10e3 3e3]  PositiveSequence=[1 0]  ExternalControl=on  NpNq=[1.3 2]  TimeConstants="[0  0  0  0]"  MinimumVoltage=0.7  Tfilter=1e-4  LoadFlowParameters=[4,0,0,0,0]
      settings: SourceProductName=Simscape Power Systems  SourceProductBaseCode=PS
  Vector Concatenate : Concatenate  Mode=Multidimensional array
  Conn1 : PMIOPort  Side=Left
  Conn2 : PMIOPort  Port=2  Side=Left
  Conn3 : PMIOPort  Port=3  Side=Left
  MPQL : Outport
  wires:
  Vector Concatenate/1 -> Three-Phase Dynamic Load/1
  Clock1/1 -> Reactive Power/1, Real Power/1
  Reactive Power/1 -> Vector Concatenate/2
  Real Power/1 -> Vector Concatenate/1
  Three-Phase Dynamic Load/1 -> MPQL/1
  connections:
  Conn1/RConn1 -- Three-Phase Dynamic Load/LConn1
  Three-Phase Dynamic Load/LConn3 -- Conn3/RConn1
  Three-Phase Dynamic Load/LConn2 -- Conn2/RConn1

== system feeder_1_1_sm_feeder1/SM_Feeder1/Dynamic Load Landfill ==
  Clock1 : Clock
  Reactive Power : Lookup_n-D  NumberOfTableDimensions=1  BreakpointsForDimension1=|  Table=|  ExtrapMethod=Clip  InternalRulePriority=Speed  RndMeth=Simplest  InputSameDT=on
      BreakpointsForDimension1=|
      | [0
      | 900
      | 1800
      | 2700
      | 3600
      | 4500
      | 5400
      | 6300
      | 7200
      | 8100
      | 9000
      | 9900
      | 10800
      | 11700
      | 12600
      | 13500
      | 14400
      | 15300
      | 16200
      | 17100
      | 18000
      | 18900
      | 19800
      | 20700
      | 21600
      | ]
      Table=|
      | [16800
      | 23952
      | 18336
      | 19872
      | 19056
      | 19056
      | 17760
      | 17088
      | 17712
      | 18768
      | 17136
      | 17616
      | 17712
      | 17328
      | 15936
      | 16896
      | 18912
      | 17616
      | 16752
      | 22320
      | 17472
      | 16800
      | 16032
      | 18576
      | 17664
      | ]
  Real Power : Lookup_n-D  NumberOfTableDimensions=1  BreakpointsForDimension1=|  Table=|  ExtrapMethod=Clip  InternalRulePriority=Speed  RndMeth=Simplest  InputSameDT=on
      BreakpointsForDimension1=|
      | [0
      | 900
      | 1800
      | 2700
      | 3600
      | 4500
      | 5400
      | 6300
      | 7200
      | 8100
      | 9000
      | 9900
      | 10800
      | 11700
      | 12600
      | 13500
      | 14400
      | 15300
      | 16200
      | 17100
      | 18000
      | 18900
      | 19800
      | 20700
      | 21600
      | ]
      Table=|
      | [27504
      | 38160
      | 37080
      | 38688
      | 37896
      | 39456
      | 37152
      | 39624
      | 38760
      | 39336
      | 39792
      | 42792
      | 40824
      | 41016
      | 39432
      | 41808
      | 45912
      | 41400
      | 40680
      | 48456
      | 41904
      | 42480
      | 39288
      | 44448
      | 42672
      | ]
  Three-Phase Dynamic Load : powerlib/Elements/Three-Phase Dynamic Load  NominalVoltage=[ 480e3 60 ]  ActiveReactivePowers=[10e3 3e3]  PositiveSequence=[1 0]  ExternalControl=on  NpNq=[1.3 2]  TimeConstants="[0  0  0  0]"  MinimumVoltage=0.7  Tfilter=1e-4  LoadFlowParameters=[4,0,0,0,0]
      settings: SourceProductName=Simscape Power Systems  SourceProductBaseCode=PS
  Vector Concatenate : Concatenate  Mode=Multidimensional array
  Conn1 : PMIOPort  Side=Left
  Conn2 : PMIOPort  Port=2  Side=Left
  Conn3 : PMIOPort  Port=3  Side=Left
  Out1 : Outport
  wires:
  Vector Concatenate/1 -> Three-Phase Dynamic Load/1
  Clock1/1 -> Reactive Power/1, Real Power/1
  Reactive Power/1 -> Vector Concatenate/2
  Real Power/1 -> Vector Concatenate/1
  Three-Phase Dynamic Load/1 -> Out1/1
  connections:
  Conn1/RConn1 -- Three-Phase Dynamic Load/LConn1
  Three-Phase Dynamic Load/LConn3 -- Conn3/RConn1
  Three-Phase Dynamic Load/LConn2 -- Conn2/RConn1

== system feeder_1_1_sm_feeder1/SM_Feeder1/PLL power injector ==
  P_ref : Inport
  "Q_ref " : Inport  Port=2
  Current Control : Subsystem
  PLL and Current  Decomposition : Subsystem
  "Power (3ph, Instantaneous)" : powerlib_meascontrol/Measurements/Power (3ph, Instantaneous)
      settings: SourceProductName=Simscape Power Systems
  SOURCES : Subsystem
  A : PMIOPort  Tag=PMCPort  Side=Right
  B : PMIOPort  Tag=PMCPort  Port=2  Side=Right
  C : PMIOPort  Tag=PMCPort  Port=3  Side=Right
  P_OUT : Outport
  Q_OUT : Outport  Port=2
  wires:
  PLL and Current  Decomposition/1(wt) -> Current Control/1(wt)
  PLL and Current  Decomposition/2(Vdq_pu) -> Current Control/2(Vdq_pu)
  PLL and Current  Decomposition/3(Idq_pu) -> Current Control/3(Idq_pu)
  Current Control/1(Vabc) -> SOURCES/1(Vabc)
  P_ref/1 -> Current Control/4(Pref)
  "Q_ref "/1 -> Current Control/5(Qref)
  "Power (3ph, Instantaneous)"/2 -> Q_OUT/1
  "Power (3ph, Instantaneous)"/1 -> P_OUT/1
  SOURCES/1(V_abc) -> PLL and Current  Decomposition/1(Vabc), "Power (3ph, Instantaneous)"/1
  SOURCES/2(I_abc) -> PLL and Current  Decomposition/2(Iabc), "Power (3ph, Instantaneous)"/2
  connections:
  A/RConn1 -- SOURCES/RConn1
  SOURCES/RConn2 -- B/RConn1
  SOURCES/RConn3 -- C/RConn1

== system feeder_1_1_sm_feeder1/SM_Feeder1/PLL power injector1 ==
  P_ref : Inport
  "Q_ref " : Inport  Port=2
  Current Control : Subsystem
  PLL and Current  Decomposition : Subsystem
  "Power (3ph, Instantaneous)" : powerlib_meascontrol/Measurements/Power (3ph, Instantaneous)
      settings: SourceProductName=Simscape Power Systems
  SOURCES : Subsystem
  A : PMIOPort  Tag=PMCPort  Side=Right
  B : PMIOPort  Tag=PMCPort  Port=2  Side=Right
  C : PMIOPort  Tag=PMCPort  Port=3  Side=Right
  P_OUT : Outport
  Q_OUT : Outport  Port=2
  wires:
  SOURCES/2(I_abc) -> "Power (3ph, Instantaneous)"/2, PLL and Current  Decomposition/2(Iabc)
  PLL and Current  Decomposition/1(wt) -> Current Control/1(wt)
  PLL and Current  Decomposition/2(Vdq_pu) -> Current Control/2(Vdq_pu)
  PLL and Current  Decomposition/3(Idq_pu) -> Current Control/3(Idq_pu)
  Current Control/1(Vabc) -> SOURCES/1(Vabc)
  P_ref/1 -> Current Control/4(Pref)
  "Q_ref "/1 -> Current Control/5(Qref)
  "Power (3ph, Instantaneous)"/2 -> Q_OUT/1
  "Power (3ph, Instantaneous)"/1 -> P_OUT/1
  SOURCES/1(V_abc) -> PLL and Current  Decomposition/1(Vabc), "Power (3ph, Instantaneous)"/1
  connections:
  A/RConn1 -- SOURCES/RConn1
  SOURCES/RConn2 -- B/RConn1
  SOURCES/RConn3 -- C/RConn1

== system feeder_1_1_sm_feeder1/SM_Feeder1/PLL power injector2 ==
  P_ref : Inport
  "Q_ref " : Inport  Port=2
  Current Control : Subsystem
  PLL and Current  Decomposition : Subsystem
  "Power (3ph, Instantaneous)" : powerlib_meascontrol/Measurements/Power (3ph, Instantaneous)
      settings: SourceProductName=Simscape Power Systems
  SOURCES : Subsystem
  A : PMIOPort  Tag=PMCPort  Side=Right
  B : PMIOPort  Tag=PMCPort  Port=2  Side=Right
  C : PMIOPort  Tag=PMCPort  Port=3  Side=Right
  P_OUT : Outport
  Q_OUT : Outport  Port=2
  wires:
  SOURCES/2(I_abc) -> "Power (3ph, Instantaneous)"/2, PLL and Current  Decomposition/2(Iabc)
  PLL and Current  Decomposition/1(wt) -> Current Control/1(wt)
  PLL and Current  Decomposition/2(Vdq_pu) -> Current Control/2(Vdq_pu)
  PLL and Current  Decomposition/3(Idq_pu) -> Current Control/3(Idq_pu)
  Current Control/1(Vabc) -> SOURCES/1(Vabc)
  P_ref/1 -> Current Control/4(Pref)
  "Q_ref "/1 -> Current Control/5(Qref)
  "Power (3ph, Instantaneous)"/2 -> Q_OUT/1
  "Power (3ph, Instantaneous)"/1 -> P_OUT/1
  SOURCES/1(V_abc) -> PLL and Current  Decomposition/1(Vabc), "Power (3ph, Instantaneous)"/1
  connections:
  A/RConn1 -- SOURCES/RConn1
  SOURCES/RConn2 -- B/RConn1
  SOURCES/RConn3 -- C/RConn1

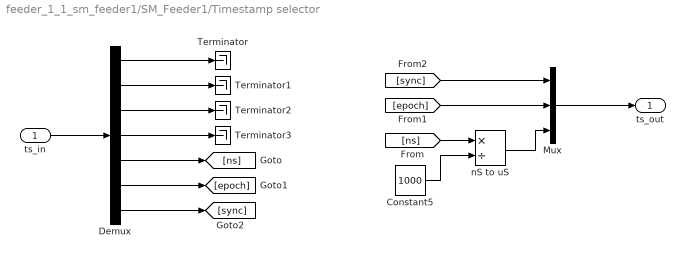
== system feeder_1_1_sm_feeder1/SM_Feeder1/Timestamp selector ==
  ts_in : Inport
  Constant5 : Constant  Value=1000
  Demux : Demux  Outputs=7
  Mux : Mux  Inputs=3
  Terminator{,1..3} (4 alike) : Terminator
  nS to uS : Product  Inputs=*/
  ts_out : Outport
  wires:
  Demux/1 -> Terminator/1
  Demux/2 -> Terminator1/1
  Demux/3 -> Terminator2/1
  Demux/4 -> Terminator3/1
  Demux/5 -> [ns]
  Demux/6 -> [epoch]
  ts_in/1 -> Demux/1
  [epoch] -> Mux/2
  Demux/7 -> [sync]
  [sync] -> Mux/1
  Mux/1 -> ts_out/1
  Constant5/1 -> nS to uS/2
  [ns] -> nS to uS/1
  nS to uS/1 -> Mux/3

== system feeder_1_1_sm_feeder1/SM_Feeder1/rtlab_send_subsystem ==
  Subsystem1 : Subsystem
  Subsystem2 : Subsystem  Priority=-200000  TreatAsAtomicUnit=on
  wires:
  [rtlab_send_1] -> Subsystem1/1(In1)
  [rtlab_send_2] -> Subsystem1/2(In2)
  [rtlab_send_5] -> Subsystem1/3(In3)
  [rtlab_send_6] -> Subsystem1/4(In4)
  [rtlab_send_7] -> Subsystem1/5(In5)
  [rtlab_send_3] -> Subsystem2/1(In1)
  [rtlab_send_4] -> Subsystem2/2(In2)
  [rtlab_send_8] -> Subsystem2/3(In3)
